simulink model "HDLRxHeader"  (R2024a)
settings: Solver=FixedStepDiscrete  StartTime=0.0  StopTime=stopTime  RelTol=1e-3
undefined symbols (not defined in the file or in its folder): CONST
libraries: dspsrcs4 x2, HDL_ieee_8021513 x2, whdledac x1
settings Model: DataTypeOverride=Off  SimulationMode=accelerator  Creator=cotti  LastModifiedBy=cotti
settings OptimizationCC: BlockReduction=off  ConditionallyExecuteInputs=off  DefaultParameterBehavior=Inlined  InheritOutputTypeSmallerThanSingle=on
settings DebuggingCC: AlgebraicLoopMsg=error  ArtificialAlgebraicLoopMsg=error  SingleTaskRateTransMsg=error  UnconnectedInputMsg=warning  UnconnectedOutputMsg=warning  UnconnectedLineMsg=warning
settings HardwareCC: ProdBitPerPointer=32  ProdBitPerSizeT=32  ProdBitPerPtrDiffT=32  ProdLargestAtomicFloat=None  ProdIntDivRoundTo=Undefined  ProdEndianess=Unspecified  ProdWordSize=32  ProdHWDeviceType=ASIC/FPGA->ASIC/FPGA  TargetBitPerLong=64  TargetBitPerPointer=64  TargetBitPerSizeT=64  TargetBitPerPtrDiffT=64  TargetLongLongMode=on  TargetIntDivRoundTo=Zero  TargetEndianess=LittleEndian  TargetWordSize=64  TargetHWDeviceType=Custom Processor->MATLAB Host Computer  ProdEqTarget=off

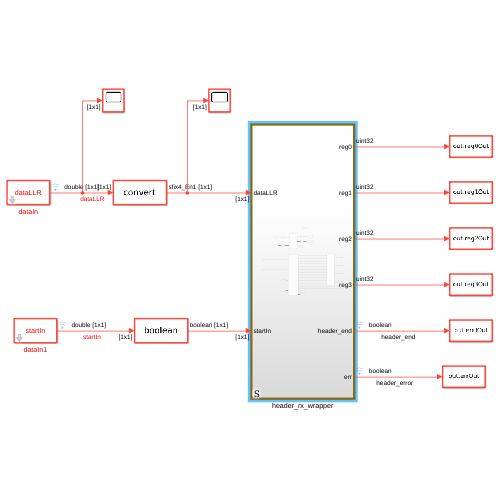
[thumbnail: Simulink's stored preview of the top-level diagram]
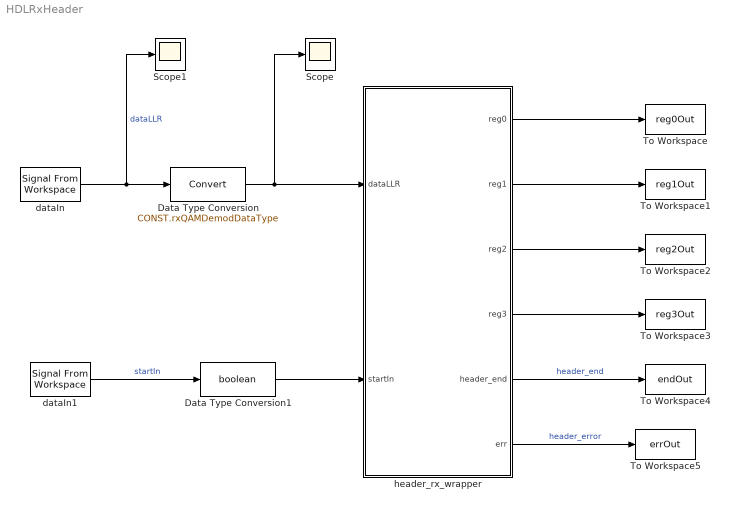
== system HDLRxHeader ==
  Data Type Conversion : DataTypeConversion  OutDataTypeStr=CONST.rxQAMDemodDataType  RndMeth=Round  SaturateOnIntegerOverflow=off
  Data Type Conversion1 : DataTypeConversion  OutDataTypeStr=boolean  SaturateOnIntegerOverflow=off  RndMeth=Floor
  Scope : Scope
  Scope1 : Scope
  To Workspace : ToWorkspace  VariableName=reg0Out  SampleTime=1/CONST.fs
      settings: Save2DSignal=2-D array (concatenate along first dimension)
  To Workspace1 : ToWorkspace  VariableName=reg1Out  SampleTime=1/CONST.fs
      settings: Save2DSignal=2-D array (concatenate along first dimension)
  To Workspace2 : ToWorkspace  VariableName=reg2Out  SampleTime=1/CONST.fs
      settings: Save2DSignal=2-D array (concatenate along first dimension)
  To Workspace3 : ToWorkspace  VariableName=reg3Out  SampleTime=1/CONST.fs
      settings: Save2DSignal=2-D array (concatenate along first dimension)
  To Workspace4 : ToWorkspace  VariableName=endOut  SampleTime=1/CONST.fs
      settings: Save2DSignal=2-D array (concatenate along first dimension)
  To Workspace5 : ToWorkspace  VariableName=errOut  SampleTime=1/CONST.fs
      settings: Save2DSignal=2-D array (concatenate along first dimension)
  dataIn : dspsrcs4/Signal From Workspace  X=dataLLR  Ts=1/CONST.fs  nsamps=1  OutputAfterFinalValue=Setting to zero  ignoreOrWarnInputAndFrameLengths=off  OutputFrames=off
  dataIn1 : dspsrcs4/Signal From Workspace  X=startIn  Ts=1/CONST.fs  nsamps=1  OutputAfterFinalValue=Setting to zero  ignoreOrWarnInputAndFrameLengths=off  OutputFrames=off
  header_rx_wrapper : Subsystem  TreatAsAtomicUnit=on
  wires:
  dataIn/1 -> Scope1/1, Data Type Conversion/1  "dataLLR"
  dataIn1/1 -> Data Type Conversion1/1  "startIn"
  header_rx_wrapper/1(reg0) -> To Workspace/1
  header_rx_wrapper/2(reg1) -> To Workspace1/1
  header_rx_wrapper/3(reg2) -> To Workspace2/1
  header_rx_wrapper/4(reg3) -> To Workspace3/1
  header_rx_wrapper/5(header_end) -> To Workspace4/1  "header_end"
  header_rx_wrapper/6(err) -> To Workspace5/1  "header_error"
  Data Type Conversion/1 -> Scope/1, header_rx_wrapper/1(dataLLR)
  Data Type Conversion1/1 -> header_rx_wrapper/2(startIn)

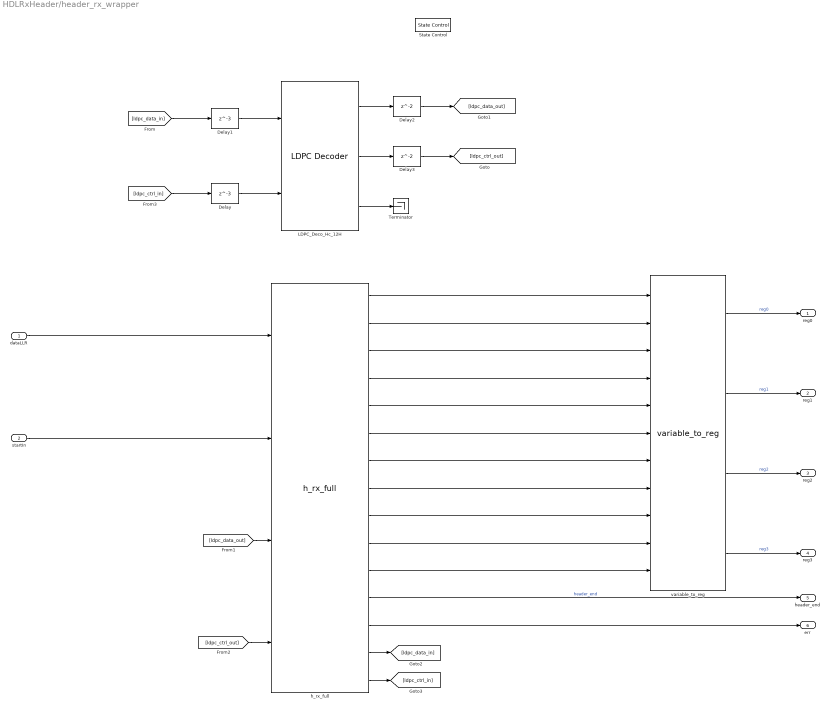
== system HDLRxHeader/header_rx_wrapper ==
  dataLLR : Inport
  startIn : Inport  Port=2
  Delay : Delay  DelayLength=3  InitialCondition=0  UseCircularBuffer=on
  Delay1 : Delay  DelayLength=3  InitialCondition=0  UseCircularBuffer=on
  Delay2 : Delay  InitialCondition=0  UseCircularBuffer=on
  Delay3 : Delay  InitialCondition=0  UseCircularBuffer=on
  LDPC_Deco_Hc_12H : whdledac/LDPC Decoder  ParityCheckMatrix=CONST.Hc_12H  BlockSize=14  Algorithm=Min-sum  ScalingFactor=0.75  Termination=Max  SpecifyInputs=Property  NumIterations=CONST.ldpcDecoderMaxNumberIterations  MaxNumIterations=8  ParityCheckStatus=off  SimulateUsing=Code generation
  State Control : StateControl  StateControl=Synchronous
  Terminator : Terminator
  h_rx_full : HDL_ieee_8021513/h_rx_full  SystemSampleTime=-1  VariantActivationTime=update diagram  AllowFlexibleInterface=on  Latency=0  AutoFrameSizeCalculation=off
      settings: SourceProductName=HDL IEEE 8021513
  variable_to_reg : HDL_ieee_8021513/variable_to_reg  SystemSampleTime=-1  VariantActivationTime=update diagram  AllowFlexibleInterface=on  Latency=0  AutoFrameSizeCalculation=off
      settings: SourceProductName=HDL IEEE 8021513
  reg0 : Outport
  reg1 : Outport  Port=2
  reg2 : Outport  Port=3
  reg3 : Outport  Port=4
  header_end : Outport  Port=5
  err : Outport  Port=6
  wires:
  Delay/1 -> LDPC_Deco_Hc_12H/2
  h_rx_full/3 -> variable_to_reg/3
  LDPC_Deco_Hc_12H/1 -> Delay2/1
  h_rx_full/5 -> variable_to_reg/5
  h_rx_full/6 -> variable_to_reg/6
  h_rx_full/10 -> variable_to_reg/10
  LDPC_Deco_Hc_12H/3 -> Terminator/1
  Delay3/1 -> [ldpc_ctrl_out]
  LDPC_Deco_Hc_12H/2 -> Delay3/1
  h_rx_full/11 -> variable_to_reg/11
  h_rx_full/4 -> variable_to_reg/4
  h_rx_full/8 -> variable_to_reg/8
  h_rx_full/12 -> header_end/1  "header_end"
  h_rx_full/1 -> variable_to_reg/1
  [ldpc_data_in] -> Delay1/1
  [ldpc_ctrl_in] -> Delay/1
  Delay2/1 -> [ldpc_data_out]
  h_rx_full/13 -> err/1
  Delay1/1 -> LDPC_Deco_Hc_12H/1
  variable_to_reg/1 -> reg0/1  "reg0"
  variable_to_reg/2 -> reg1/1  "reg1"
  [ldpc_ctrl_out] -> h_rx_full/4
  h_rx_full/14 -> [ldpc_data_in]
  [ldpc_data_out] -> h_rx_full/3
  variable_to_reg/3 -> reg2/1  "reg2"
  dataLLR/1 -> h_rx_full/1
  h_rx_full/15 -> [ldpc_ctrl_in]
  startIn/1 -> h_rx_full/2
  h_rx_full/9 -> variable_to_reg/9
  variable_to_reg/4 -> reg3/1  "reg3"
  h_rx_full/2 -> variable_to_reg/2
  h_rx_full/7 -> variable_to_reg/7
